simulink model "eBikeDigitalTwin"  (R2023b)
settings: Solver=VariableStepAuto  StartTime=0.0  StopTime=10.0  RelTol=1e-3
libraries: ee_lib x14, fl_lib x7, batteryecm_lib x4, spsPermanentMagnetSynchronousMachineLib x1
settings Model: Creator=epier  LastModifiedBy=epier

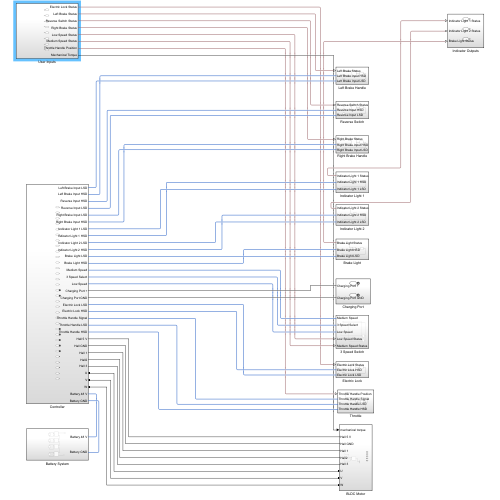
[thumbnail: Simulink's stored preview of the top-level diagram]
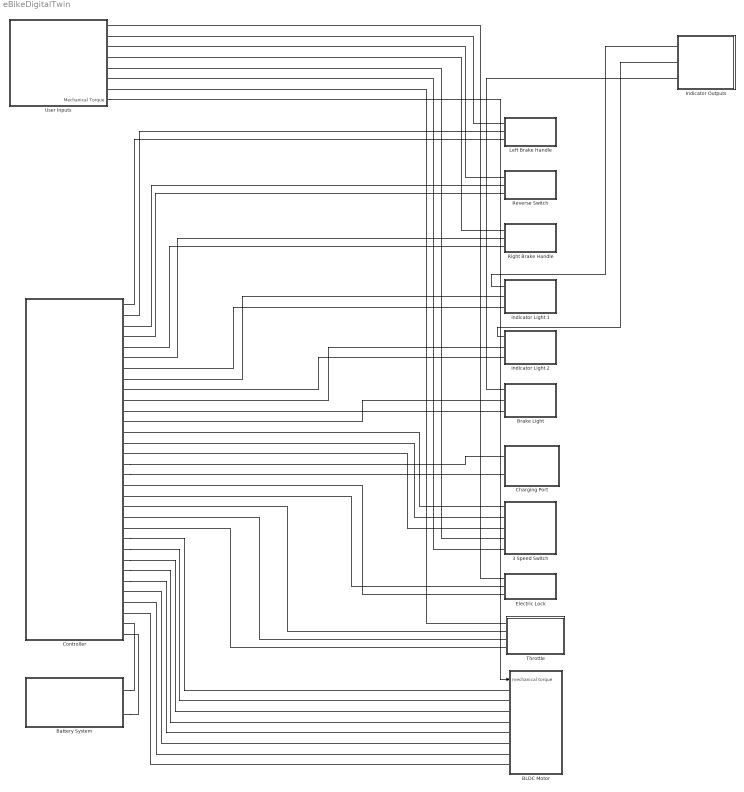
== system eBikeDigitalTwin ==
  3 Speed Switch : Subsystem
  BLDC Motor : Subsystem
      settings: PortSchema="{\"entries\":[{\"content\":{\"sides\":[{\"content\":{},\"type\":\"ConnectorPlacement.EquallySpacedRectSide\",\"uuid\":\"6f305cfd-3a6e-4ac1-8ccb-5bca266a502d\"},{\"content\":{\"connectorIds\":[\"In1\",\"RConn1\",\"RConn2\",\"RConn3\",\"RConn4\",\"RConn5\",\"RConn6\",\"RConn7\",\"RConn8\"],\"side\":\"RIGHT\"},\"type\":\"ConnectorPlacement.EquallySpacedRectSide\",\"uuid\":\"3c37ef43-0ddf-4dcc-b8e6-a30a230bdb34\"},{\"content\":{\"side\":\"TOP\"},\"type\":\"ConnectorPlacement.EquallySpacedRectSide\",\"uuid\":\"8af75aaf-b5e7-47d0-9c7f-87a962c63755\"}]},\"type\":\"ConnectorPlacement.EquallySpacedConnector\",\"uuid\":\"baf254ef-54e0-4d0e-9512-c63c4e1739b8\"}],\"packageUris\":[\"http://schema.mathworks.com/mf0/Connector/R2020b\"],\"version\":\"1.0\"}"
  Battery System : Subsystem
  Brake Light : Subsystem
  Charging Port : Subsystem
  Controller : Subsystem
  Electric Lock : Subsystem
  Indicator Light 1 : Subsystem
  Indicator Light 2 : Subsystem
  Indicator Outputs : Subsystem
  Left Brake Handle : Subsystem
  Reverse Switch : Subsystem
  Right Brake Handle : Subsystem
  Throttle : Subsystem
  User Inputs : Subsystem
      settings: PortSchema="{\"entries\":[{\"content\":{\"sides\":[{\"content\":{},\"type\":\"ConnectorPlacement.EquallySpacedRectSide\",\"uuid\":\"c4874808-4bc0-4391-ab50-9ee5c3ad01f9\"},{\"content\":{\"connectorIds\":[\"RConn1\",\"RConn2\",\"RConn3\",\"RConn4\",\"RConn5\",\"RConn6\",\"RConn7\",\"Out1\"],\"side\":\"RIGHT\"},\"type\":\"ConnectorPlacement.EquallySpacedRectSide\",\"uuid\":\"5fcb0844-4dd2-4d4a-9281-d992b8247c18\"},{\"content\":{\"side\":\"TOP\"},\"type\":\"ConnectorPlacement.EquallySpacedRectSide\",\"uuid\":\"f8d96913-3646-41c7-98dc-9e2b9fe885e6\"}]},\"type\":\"ConnectorPlacement.EquallySpacedConnector\",\"uuid\":\"3c384b36-bf68-40a4-b8b5-a19355291a85\"}],\"packageUris\":[\"http://schema.mathworks.com/mf0/Connector/R2020b\"],\"version\":\"1.0\"}"
  wires:
  User Inputs/1(Mechanical Torque) -> BLDC Motor/1(mechanical torque)
  connections:
  Electric Lock/LConn1 -- User Inputs/RConn1
  Left Brake Handle/LConn1 -- User Inputs/RConn2
  Reverse Switch/LConn1 -- User Inputs/RConn3
  Right Brake Handle/LConn1 -- User Inputs/RConn4
  Left Brake Handle/LConn2 -- Controller/LConn2
  Left Brake Handle/LConn3 -- Controller/LConn1
  Reverse Switch/LConn2 -- Controller/LConn3
  Reverse Switch/LConn3 -- Controller/LConn4
  Right Brake Handle/LConn3 -- Controller/LConn5
  Right Brake Handle/LConn2 -- Controller/LConn6
  Indicator Light 1/LConn1 -- Indicator Outputs/LConn1
  Indicator Light 1/LConn3 -- Controller/LConn7
  Indicator Light 1/LConn2 -- Controller/LConn8
  Indicator Light 2/LConn1 -- Indicator Outputs/LConn2
  Indicator Light 2/LConn3 -- Controller/LConn9
  Indicator Light 2/LConn2 -- Controller/LConn10
  Brake Light/LConn1 -- Indicator Outputs/LConn3
  Brake Light/LConn3 -- Controller/LConn11
  Brake Light/LConn2 -- Controller/LConn12
  3 Speed Switch/LConn4 -- User Inputs/RConn5
  3 Speed Switch/LConn5 -- User Inputs/RConn6
  3 Speed Switch/LConn1 -- Controller/LConn13
  3 Speed Switch/LConn2 -- Controller/LConn14
  3 Speed Switch/LConn3 -- Controller/LConn15
  Electric Lock/LConn3 -- Controller/LConn18
  Electric Lock/LConn2 -- Controller/LConn19
  Throttle/LConn1 -- User Inputs/RConn7
  Throttle/LConn2 -- Controller/LConn20
  Throttle/LConn3 -- Controller/LConn21
  Throttle/LConn4 -- Controller/LConn22
  BLDC Motor/RConn6 -- Controller/LConn28
  BLDC Motor/RConn7 -- Controller/LConn29
  BLDC Motor/RConn8 -- Controller/LConn30
  Controller/LConn23 -- BLDC Motor/RConn1
  Controller/LConn24 -- BLDC Motor/RConn2
  Controller/LConn25 -- BLDC Motor/RConn3
  Controller/LConn26 -- BLDC Motor/RConn4
  Controller/LConn27 -- BLDC Motor/RConn5
  Controller/LConn16 -- Charging Port/LConn1
  Controller/LConn17 -- Charging Port/LConn2
  Battery System/RConn1 -- Controller/LConn31
  Battery System/RConn2 -- Controller/LConn32

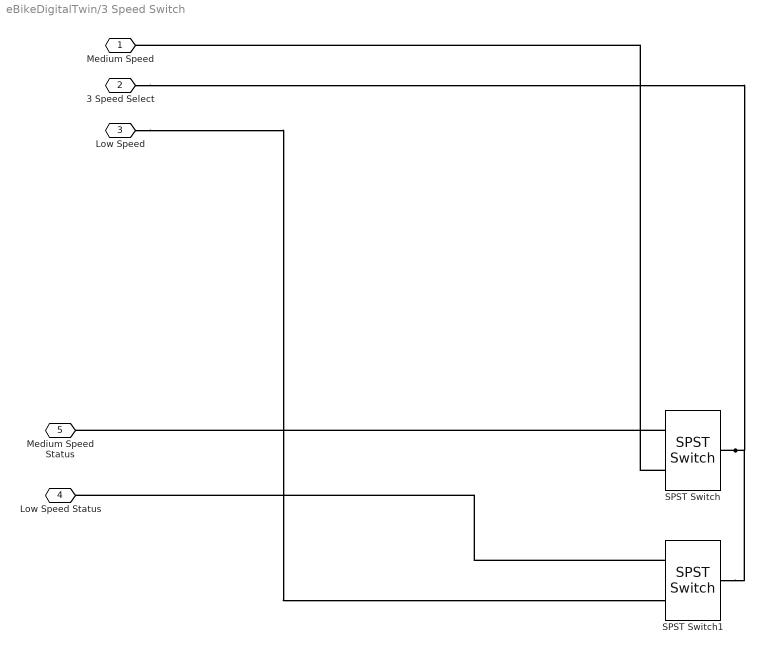
== system eBikeDigitalTwin/3 Speed Switch ==
  SPST Switch : ee_lib/Switches & Breakers/SPST Switch  R_closed=0.01 Ohm  G_open=1e-6 S  Threshold=0.5 V  Width=0 V  model_dynamics=0  t_on=1e-3 s  t_off=1e-3 s  initial_vT=0 V
      settings: InternalSimscapePortConfiguration="{\"Bottom\":[],\"Left\":[{\"id\":\"vT\",\"label\":\"vT\",\"type\":\"input\"},{\"id\":\"p\",\"label\":\"\",\"type\":\"foundation.electrical.electrical\"}],\"Right\":[{\"id\":\"n\",\"label\":\"\",\"type\":\"foundation.electrical.electrical\"}],\"Top\":[]}"
  SPST Switch1 : ee_lib/Switches & Breakers/SPST Switch  R_closed=0.01 Ohm  G_open=1e-6 S  Threshold=0.5 V  Width=0 V  model_dynamics=0  t_on=1e-3 s  t_off=1e-3 s  initial_vT=0 V
      settings: InternalSimscapePortConfiguration="{\"Bottom\":[],\"Left\":[{\"id\":\"vT\",\"label\":\"vT\",\"type\":\"input\"},{\"id\":\"p\",\"label\":\"\",\"type\":\"foundation.electrical.electrical\"}],\"Right\":[{\"id\":\"n\",\"label\":\"\",\"type\":\"foundation.electrical.electrical\"}],\"Top\":[]}"
  Medium Speed : PMIOPort  Side=Left
  3 Speed Select : PMIOPort  Port=2  Side=Left
  Low Speed : PMIOPort  Port=3  Side=Left
  Low Speed Status : PMIOPort  Port=4  Side=Left
  Medium Speed Status : PMIOPort  Port=5  Side=Left
  connections:
  SPST Switch/RConn1 -- 3 Speed Select/RConn1 -- SPST Switch1/RConn1
  SPST Switch1/LConn1 -- Low Speed Status/RConn1
  Low Speed/RConn1 -- SPST Switch1/LConn2
  SPST Switch/LConn1 -- Medium Speed Status/RConn1
  SPST Switch/LConn2 -- Medium Speed/RConn1

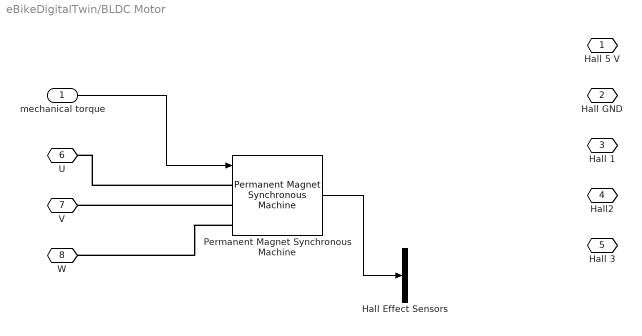
== system eBikeDigitalTwin/BLDC Motor ==
  mechanical torque : Inport
  Hall Effect Sensors : Demux  Outputs=3
  Permanent Magnet Synchronous Machine : spsPermanentMagnetSynchronousMachineLib/Permanent Magnet Synchronous Machine  NbPhases=3  FluxDistribution=Sinusoidal  RotorType=Round  MechanicalLoad=Torque Tm  PresetModel=No  ShowDetailedParameters=on  MeasurementBus=off  Resistance=0.0485  Inductance=8.5e-3  dqInductances=[8.5e-3,8.5e-3]  La=0.000395  MachineConstant=Flux linkage established by magnets (V.s)  Flux=0.1194  VoltageCst=86.6271  TorqueCst=0.7164  Flat=120  Mechanical=[0.0027 0.0004924 4 0]  PolePairs=4  InitialConditions=[0,0, 0,0]  InitialConditions5ph=[0 0 0 0 0 0]  RefAngle=90 degrees behind phase A axis (modified Park)  IterativeDiscreteModel=Trapezoidal non iterative  TsBlock=-1  TsPowergui=0
  Hall 5 V : PMIOPort  Side=Right
  Hall GND : PMIOPort  Port=2  Side=Right
  Hall 1 : PMIOPort  Port=3  Side=Right
  Hall2 : PMIOPort  Port=4  Side=Right
  Hall 3 : PMIOPort  Port=5  Side=Right
  U : PMIOPort  Port=6  Side=Right
  V : PMIOPort  Port=7  Side=Right
  W : PMIOPort  Port=8  Side=Right
  wires:
  Permanent Magnet Synchronous Machine/1 -> Hall Effect Sensors/1
  mechanical torque/1 -> Permanent Magnet Synchronous Machine/1
  connections:
  Permanent Magnet Synchronous Machine/LConn1 -- U/RConn1
  Permanent Magnet Synchronous Machine/LConn2 -- V/RConn1
  Permanent Magnet Synchronous Machine/LConn3 -- W/RConn1

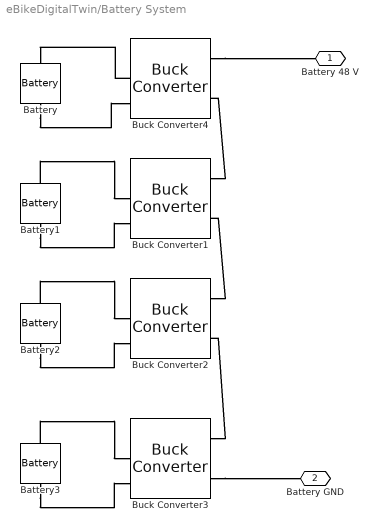
== system eBikeDigitalTwin/Battery System ==
  Battery{,1..3} (4 alike) : batteryecm_lib/Battery  Vnom=12 V  prm_dir=simscape.enum.battery.prm_dir.disabled  R1_dis=2 Ohm  R1_ch=2 Ohm  R1=2 Ohm  prm_AH=simscape.enum.battery.prm_AH.infinite  AH=50 A*hr  V1=11.5 V  AH1=25 A*hr  prm_R2=simscape.enum.battery.prm_R2.disabled  R2=2000 Ohm  Tmeas=298.15 K  charge_measurement_port=simscape.enum.battery.enable.no  prm_dyn=simscape.enum.battery.prm_dyn.off  Rp1=0.005 Ohm  tau1=30 s  Rp2=0.005 Ohm  tau2=30 s  Rp3=0.005 Ohm  tau3=30 s  Rp4=0.005 Ohm  tau4=30 s  Rp5=0.005 Ohm  tau5=30 s  prm_fade=simscape.enum.battery.prm_fade.disabled  N_fade=100  AH_fade=45 A*hr  R1_fade=2.02 Ohm  R1_ch_fade=2.02 Ohm  V1_fade=10.35 V  prm_age=simscape.enum.battery.prm_age.disabled  prm_age_OCV=simscape.enum.battery.prm_age_OCV.OCV  OCV_age=0.9  SOC_age=60  Tmeas_age=298.15 K  delta_time_age_vec=[0] d  temperature_age_vec=[273] K  OCV_scaling_age=2.2134e6  OCV_offset_age=1.632e6  temp_exp_age=0.515833569 V  t_exp_age=0.75  Vnom_T2=12 V  R1_T2=2.2 Ohm  R1_T2_dis=2.2 Ohm  R1_T2_ch=2.2 Ohm  V1_T2=11.4 V  R2_T2=2200 Ohm  Rp1_T2=0.005 Ohm  tau1_T2=30 s  Rp2_T2=0.005 Ohm  tau2_T2=30 s  Rp3_T2=0.005 Ohm  tau3_T2=30 s  Rp4_T2=0.005 Ohm  tau4_T2=30 s  Rp5_T2=0.005 Ohm  tau5_T2=30 s  Tmeas2=273.15 K  thermal_port=simscape.enum.thermaleffects.omit  thermal_mass=30000 J/K  i_specify=off  i_priority=None  i=0 A  i_nominal_specify=off  i_nominal_unit=A  i_nominal_value=1  v_specify=off  v_priority=None  v=0 V  v_nominal_specify=off  v_nominal_unit=V  v_nominal_value=1  charge_specify=off  charge_priority=High  charge=50 A*hr  charge_nominal_specify=off  charge_nominal_unit=A*hr  charge_nominal_value=1  num_cycles_specify=off  num_cycles_priority=High  num_cycles=0  num_cycles_nominal_specify=off  num_cycles_nominal_unit=1  num_cycles_nominal_value=1  temperature_specify=off  temperature_priority=High  temperature=298.15 K  temperature_nominal_specify=off  temperature_nominal_unit=K  temperature_nominal_value=1
  Buck Converter{1..4} (4 alike) : ee_lib/Semiconductors & Converters/Converters/Buck Converter  port_option=ee.enum.controlport.ps  device_type=ee.enum.converters.switchingdevice.ideal  Vf=0.8 V  Ron=0.001 Ohm  Rds=0.001 Ohm  Goff=1e-5 1/Ohm  Vgt=1 V  Vgt_off=-1 V  Ih=1 A  Vth=12 V  K=0  diode_param=ee.enum.converters.protectiondiode.nodynamics  diode_Vf=0.8 V  diode_Ron=0.001 Ohm  diode_Goff=1e-5 1/Ohm  diode_C=50 nF  diode_iRM=-235 A  diode_iF=300 A  diode_idot=-50 A/us  diode_trr_param=ee.enum.converters.diodetrr.trr_factor  diode_trr_factor=3  diode_trr=15 us  diode_Qrr=1500 s*uA  Lf=1e-6 H  Rl=0 Ohm  Cf=1e-7 F  Rf=1e-6 Ohm  snubber_type=ee.enum.converters.snubber.exclude  Cs=1e-7 F  Rs=0.1 Ohm  iL_specify=off  iL_priority=High  iL=0 A  iL_nominal_specify=off  iL_nominal_unit=A  iL_nominal_value=1  vc_specify=off  vc_priority=High  vc=0 V  vc_nominal_specify=off  vc_nominal_unit=V  vc_nominal_value=1
      settings: InternalSimscapePortConfiguration="{\"Bottom\":[],\"Left\":[{\"id\":\"G\",\"label\":\"G\",\"type\":\"input\"},{\"id\":\"p1\",\"label\":\"1+\",\"type\":\"foundation.electrical.electrical\"},{\"id\":\"n1\",\"label\":\"1-\",\"type\":\"foundation.electrical.electrical\"}],\"Right\":[{\"id\":\"p2\",\"label\":\"2+\",\"type\":\"foundation.electrical.electrical\"},{\"id\":\"n2\",\"label\":\"2-\",\"type\":\"foundation.electrical.electrical\"}],\"Top\":[]}"
  Battery 48 V : PMIOPort  Side=Right
  Battery GND : PMIOPort  Port=2  Side=Right
  connections:
  Buck Converter4/LConn2 -- Battery/LConn1
  Battery1/LConn1 -- Buck Converter1/LConn2
  Battery/RConn1 -- Buck Converter4/LConn3
  Buck Converter4/RConn1 -- Battery 48 V/RConn1
  Battery1/RConn1 -- Buck Converter1/LConn3
  Battery2/RConn1 -- Buck Converter2/LConn3
  Battery2/LConn1 -- Buck Converter2/LConn2
  Battery3/RConn1 -- Buck Converter3/LConn3
  Battery3/LConn1 -- Buck Converter3/LConn2
  Buck Converter3/RConn2 -- Battery GND/RConn1
  Buck Converter3/RConn1 -- Buck Converter2/RConn2
  Buck Converter2/RConn1 -- Buck Converter1/RConn2
  Buck Converter1/RConn1 -- Buck Converter4/RConn2

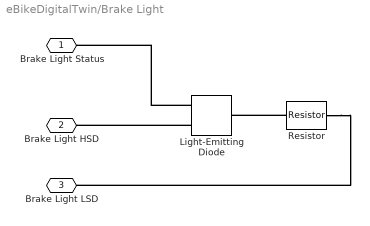
== system eBikeDigitalTwin/Brake Light ==
  Light-Emitting Diode : ee_lib/Sensors & Transducers/Light-Emitting Diode  Gain=0.005 W/A  prmExp=1  I12=[.0017, .003] A  V12=[.9, 1.05] V  IS=5e-5 A  ec=10  RS=0.1 Ohm  Tmeas=25 degC  C_param=1  CJ=20 pF  CJ0=20 pF  VJ=1 V  Mgrad=0.5  Vvec=[.1, 10, 100] V  Cvec=[15, 10, 2] pF  FC=0.5  T_param=1  IS_T2=1.8e-4 A  I1_T2=0.0034 A  V1_T2=1.05 V  Tmeas2=125 degC  EG_param=1  EG=1.11 eV  XTI_param=1  XTI=3  Tdevice=25 degC  i_specify=off  i_priority=None  i=0 A  i_nominal_specify=off  i_nominal_unit=A  i_nominal_value=1  v_specify=off  v_priority=None  v=0 V  v_nominal_specify=off  v_nominal_unit=V  v_nominal_value=1  v_capacitor_specify=off  v_capacitor_priority=High  v_capacitor=0 V  v_capacitor_nominal_specify=off  v_capacitor_nominal_unit=V  v_capacitor_nominal_value=1  thermal_network_parameterization=ee.enum.thermalNetworkTopology.junctionCase  Rth=[0, 10] K/W  Rth_Cauer=[1, 3, 10] K/W  Rth_Foster=[4, 6] K/W  thermal_mass_parameterization=ee.enum.thermalNetwork.timeconstant  thermal_mass=[0, 1] J/K  thermal_mass_Cauer=[1.5, 2, 3] J/K  thermal_mass_Foster=[1.5, 3] J/K  thermal_time_constant=[0, 10] s  thermal_time_constant_Cauer=[1, 3, 10] s  thermal_time_constant_Foster=[6, 18] s  thermal_mass_initial_temperatures=[25, 25] degC  thermal_mass_initial_temperatures_Cauer=[25, 25, 25] degC  steadyState_Foster=simscape.enum.onoff.on  Tvec_initial_Foster=[25, 25, 25, 25] degC
      settings: InternalSimscapePortConfiguration="{\"Bottom\":[],\"Left\":[{\"id\":\"W\",\"label\":\"W\",\"type\":\"output\"},{\"id\":\"p\",\"label\":\"\",\"type\":\"foundation.electrical.electrical\"}],\"Right\":[{\"id\":\"n\",\"label\":\"\",\"type\":\"foundation.electrical.electrical\"}],\"Top\":[]}"
  Resistor : fl_lib/Electrical/Electrical Elements/Resistor  R=1 Ohm  i_specify=off  i_priority=None  i=0 A  i_nominal_specify=off  i_nominal_unit=A  i_nominal_value=1  v_specify=off  v_priority=None  v=0 V  v_nominal_specify=off  v_nominal_unit=V  v_nominal_value=1
  Brake Light Status : PMIOPort  Side=Left
  Brake Light HSD : PMIOPort  Port=2  Side=Left
  Brake Light LSD : PMIOPort  Port=3  Side=Left
  connections:
  Light-Emitting Diode/LConn1 -- Brake Light Status/RConn1
  Resistor/RConn1 -- Brake Light LSD/RConn1
  Resistor/LConn1 -- Light-Emitting Diode/RConn1
  Light-Emitting Diode/LConn2 -- Brake Light HSD/RConn1

== system eBikeDigitalTwin/Charging Port ==
  Charging Port + : PMIOPort  Side=Left
  Charging Port GND : PMIOPort  Port=2  Side=Left

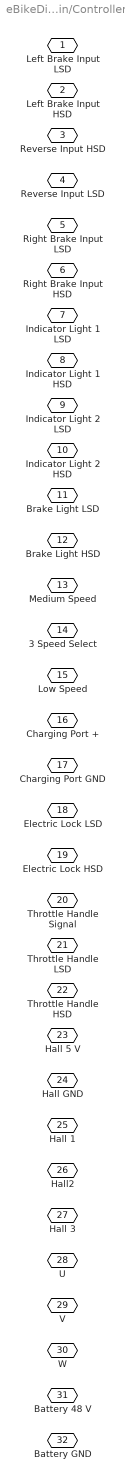
== system eBikeDigitalTwin/Controller ==
  Left Brake Input LSD : PMIOPort  Side=Left
  Left Brake Input HSD : PMIOPort  Port=2  Side=Left
  Reverse Input HSD : PMIOPort  Port=3  Side=Left
  Reverse Input LSD : PMIOPort  Port=4  Side=Left
  Right Brake Input LSD : PMIOPort  Port=5  Side=Left
  Right Brake Input HSD : PMIOPort  Port=6  Side=Left
  Indicator Light 1 LSD : PMIOPort  Port=7  Side=Left
  Indicator Light 1 HSD : PMIOPort  Port=8  Side=Left
  Indicator Light 2 LSD : PMIOPort  Port=9  Side=Left
  Indicator Light 2 HSD : PMIOPort  Port=10  Side=Left
  Brake Light LSD : PMIOPort  Port=11  Side=Left
  Brake Light HSD : PMIOPort  Port=12  Side=Left
  Medium Speed : PMIOPort  Port=13  Side=Left
  3 Speed Select : PMIOPort  Port=14  Side=Left
  Low Speed : PMIOPort  Port=15  Side=Left
  Charging Port + : PMIOPort  Port=16  Side=Left
  Charging Port GND : PMIOPort  Port=17  Side=Left
  Electric Lock LSD : PMIOPort  Port=18  Side=Left
  Electric Lock HSD : PMIOPort  Port=19  Side=Left
  Throttle Handle Signal : PMIOPort  Port=20  Side=Left
  Throttle Handle LSD : PMIOPort  Port=21  Side=Left
  Throttle Handle HSD : PMIOPort  Port=22  Side=Left
  Hall 5 V : PMIOPort  Port=23  Side=Left
  Hall GND : PMIOPort  Port=24  Side=Left
  Hall 1 : PMIOPort  Port=25  Side=Left
  Hall2 : PMIOPort  Port=26  Side=Left
  Hall 3 : PMIOPort  Port=27  Side=Left
  U : PMIOPort  Port=28  Side=Left
  V : PMIOPort  Port=29  Side=Left
  W : PMIOPort  Port=30  Side=Left
  Battery 48 V : PMIOPort  Port=31  Side=Left
  Battery GND : PMIOPort  Port=32  Side=Left

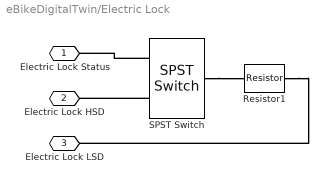
== system eBikeDigitalTwin/Electric Lock ==
  Resistor1 : fl_lib/Electrical/Electrical Elements/Resistor  R=0.8 Ohm  i_specify=off  i_priority=None  i=0 A  i_nominal_specify=off  i_nominal_unit=A  i_nominal_value=1  v_specify=off  v_priority=None  v=0 V  v_nominal_specify=off  v_nominal_unit=V  v_nominal_value=1
  SPST Switch : ee_lib/Switches & Breakers/SPST Switch  R_closed=0.01 Ohm  G_open=1e-6 S  Threshold=0.5 V  Width=0 V  model_dynamics=0  t_on=1e-3 s  t_off=1e-3 s  initial_vT=0 V
      settings: InternalSimscapePortConfiguration="{\"Bottom\":[],\"Left\":[{\"id\":\"vT\",\"label\":\"vT\",\"type\":\"input\"},{\"id\":\"p\",\"label\":\"\",\"type\":\"foundation.electrical.electrical\"}],\"Right\":[{\"id\":\"n\",\"label\":\"\",\"type\":\"foundation.electrical.electrical\"}],\"Top\":[]}"
  Electric Lock Status : PMIOPort  Side=Left
  Electric Lock HSD : PMIOPort  Port=2  Side=Left
  Electric Lock LSD : PMIOPort  Port=3  Side=Left
  connections:
  SPST Switch/RConn1 -- Resistor1/LConn1
  SPST Switch/LConn1 -- Electric Lock Status/RConn1
  Resistor1/RConn1 -- Electric Lock LSD/RConn1
  SPST Switch/LConn2 -- Electric Lock HSD/RConn1

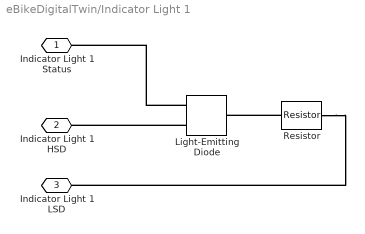
== system eBikeDigitalTwin/Indicator Light 1 ==
  Light-Emitting Diode : ee_lib/Sensors & Transducers/Light-Emitting Diode  Gain=0.005 W/A  prmExp=1  I12=[.0017, .003] A  V12=[.9, 1.05] V  IS=5e-5 A  ec=10  RS=0.1 Ohm  Tmeas=25 degC  C_param=1  CJ=20 pF  CJ0=20 pF  VJ=1 V  Mgrad=0.5  Vvec=[.1, 10, 100] V  Cvec=[15, 10, 2] pF  FC=0.5  T_param=1  IS_T2=1.8e-4 A  I1_T2=0.0034 A  V1_T2=1.05 V  Tmeas2=125 degC  EG_param=1  EG=1.11 eV  XTI_param=1  XTI=3  Tdevice=25 degC  i_specify=off  i_priority=None  i=0 A  i_nominal_specify=off  i_nominal_unit=A  i_nominal_value=1  v_specify=off  v_priority=None  v=0 V  v_nominal_specify=off  v_nominal_unit=V  v_nominal_value=1  v_capacitor_specify=off  v_capacitor_priority=High  v_capacitor=0 V  v_capacitor_nominal_specify=off  v_capacitor_nominal_unit=V  v_capacitor_nominal_value=1  thermal_network_parameterization=ee.enum.thermalNetworkTopology.junctionCase  Rth=[0, 10] K/W  Rth_Cauer=[1, 3, 10] K/W  Rth_Foster=[4, 6] K/W  thermal_mass_parameterization=ee.enum.thermalNetwork.timeconstant  thermal_mass=[0, 1] J/K  thermal_mass_Cauer=[1.5, 2, 3] J/K  thermal_mass_Foster=[1.5, 3] J/K  thermal_time_constant=[0, 10] s  thermal_time_constant_Cauer=[1, 3, 10] s  thermal_time_constant_Foster=[6, 18] s  thermal_mass_initial_temperatures=[25, 25] degC  thermal_mass_initial_temperatures_Cauer=[25, 25, 25] degC  steadyState_Foster=simscape.enum.onoff.on  Tvec_initial_Foster=[25, 25, 25, 25] degC
      settings: InternalSimscapePortConfiguration="{\"Bottom\":[],\"Left\":[{\"id\":\"W\",\"label\":\"W\",\"type\":\"output\"},{\"id\":\"p\",\"label\":\"\",\"type\":\"foundation.electrical.electrical\"}],\"Right\":[{\"id\":\"n\",\"label\":\"\",\"type\":\"foundation.electrical.electrical\"}],\"Top\":[]}"
  Resistor : fl_lib/Electrical/Electrical Elements/Resistor  R=1 Ohm  i_specify=off  i_priority=None  i=0 A  i_nominal_specify=off  i_nominal_unit=A  i_nominal_value=1  v_specify=off  v_priority=None  v=0 V  v_nominal_specify=off  v_nominal_unit=V  v_nominal_value=1
  Indicator Light 1 Status : PMIOPort  Side=Left
  Indicator Light 1 HSD : PMIOPort  Port=2  Side=Left
  Indicator Light 1 LSD : PMIOPort  Port=3  Side=Left
  connections:
  Light-Emitting Diode/LConn1 -- Indicator Light 1 Status/RConn1
  Resistor/RConn1 -- Indicator Light 1 LSD/RConn1
  Resistor/LConn1 -- Light-Emitting Diode/RConn1
  Light-Emitting Diode/LConn2 -- Indicator Light 1 HSD/RConn1

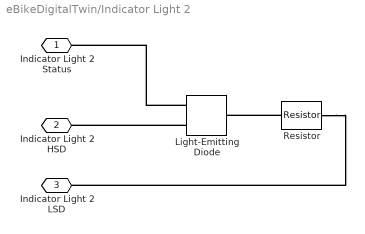
== system eBikeDigitalTwin/Indicator Light 2 ==
  Light-Emitting Diode : ee_lib/Sensors & Transducers/Light-Emitting Diode  Gain=0.005 W/A  prmExp=1  I12=[.0017, .003] A  V12=[.9, 1.05] V  IS=5e-5 A  ec=10  RS=0.1 Ohm  Tmeas=25 degC  C_param=1  CJ=20 pF  CJ0=20 pF  VJ=1 V  Mgrad=0.5  Vvec=[.1, 10, 100] V  Cvec=[15, 10, 2] pF  FC=0.5  T_param=1  IS_T2=1.8e-4 A  I1_T2=0.0034 A  V1_T2=1.05 V  Tmeas2=125 degC  EG_param=1  EG=1.11 eV  XTI_param=1  XTI=3  Tdevice=25 degC  i_specify=off  i_priority=None  i=0 A  i_nominal_specify=off  i_nominal_unit=A  i_nominal_value=1  v_specify=off  v_priority=None  v=0 V  v_nominal_specify=off  v_nominal_unit=V  v_nominal_value=1  v_capacitor_specify=off  v_capacitor_priority=High  v_capacitor=0 V  v_capacitor_nominal_specify=off  v_capacitor_nominal_unit=V  v_capacitor_nominal_value=1  thermal_network_parameterization=ee.enum.thermalNetworkTopology.junctionCase  Rth=[0, 10] K/W  Rth_Cauer=[1, 3, 10] K/W  Rth_Foster=[4, 6] K/W  thermal_mass_parameterization=ee.enum.thermalNetwork.timeconstant  thermal_mass=[0, 1] J/K  thermal_mass_Cauer=[1.5, 2, 3] J/K  thermal_mass_Foster=[1.5, 3] J/K  thermal_time_constant=[0, 10] s  thermal_time_constant_Cauer=[1, 3, 10] s  thermal_time_constant_Foster=[6, 18] s  thermal_mass_initial_temperatures=[25, 25] degC  thermal_mass_initial_temperatures_Cauer=[25, 25, 25] degC  steadyState_Foster=simscape.enum.onoff.on  Tvec_initial_Foster=[25, 25, 25, 25] degC
      settings: InternalSimscapePortConfiguration="{\"Bottom\":[],\"Left\":[{\"id\":\"W\",\"label\":\"W\",\"type\":\"output\"},{\"id\":\"p\",\"label\":\"\",\"type\":\"foundation.electrical.electrical\"}],\"Right\":[{\"id\":\"n\",\"label\":\"\",\"type\":\"foundation.electrical.electrical\"}],\"Top\":[]}"
  Resistor : fl_lib/Electrical/Electrical Elements/Resistor  R=1 Ohm  i_specify=off  i_priority=None  i=0 A  i_nominal_specify=off  i_nominal_unit=A  i_nominal_value=1  v_specify=off  v_priority=None  v=0 V  v_nominal_specify=off  v_nominal_unit=V  v_nominal_value=1
  Indicator Light 2 Status : PMIOPort  Side=Left
  Indicator Light 2 HSD : PMIOPort  Port=2  Side=Left
  Indicator Light 2 LSD : PMIOPort  Port=3  Side=Left
  connections:
  Light-Emitting Diode/LConn1 -- Indicator Light 2 Status/RConn1
  Resistor/RConn1 -- Indicator Light 2 LSD/RConn1
  Resistor/LConn1 -- Light-Emitting Diode/RConn1
  Light-Emitting Diode/LConn2 -- Indicator Light 2 HSD/RConn1

== system eBikeDigitalTwin/Indicator Outputs ==
  Indicator Light 1 Status : PMIOPort  Side=Left
  Indicator Light 2 Status : PMIOPort  Port=2  Side=Left
  Brake Light Status : PMIOPort  Port=3  Side=Left

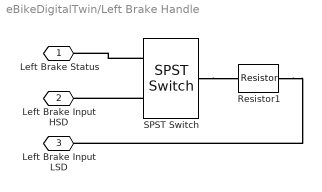
== system eBikeDigitalTwin/Left Brake Handle ==
  Resistor1 : fl_lib/Electrical/Electrical Elements/Resistor  R=0.8 Ohm  i_specify=off  i_priority=None  i=0 A  i_nominal_specify=off  i_nominal_unit=A  i_nominal_value=1  v_specify=off  v_priority=None  v=0 V  v_nominal_specify=off  v_nominal_unit=V  v_nominal_value=1
  SPST Switch : ee_lib/Switches & Breakers/SPST Switch  R_closed=0.01 Ohm  G_open=1e-6 S  Threshold=0.5 V  Width=0 V  model_dynamics=0  t_on=1e-3 s  t_off=1e-3 s  initial_vT=0 V
      settings: InternalSimscapePortConfiguration="{\"Bottom\":[],\"Left\":[{\"id\":\"vT\",\"label\":\"vT\",\"type\":\"input\"},{\"id\":\"p\",\"label\":\"\",\"type\":\"foundation.electrical.electrical\"}],\"Right\":[{\"id\":\"n\",\"label\":\"\",\"type\":\"foundation.electrical.electrical\"}],\"Top\":[]}"
  Left Brake Status : PMIOPort  Side=Left
  Left Brake Input HSD : PMIOPort  Port=2  Side=Left
  Left Brake Input LSD : PMIOPort  Port=3  Side=Left
  connections:
  SPST Switch/RConn1 -- Resistor1/LConn1
  SPST Switch/LConn1 -- Left Brake Status/RConn1
  Resistor1/RConn1 -- Left Brake Input LSD/RConn1
  SPST Switch/LConn2 -- Left Brake Input HSD/RConn1

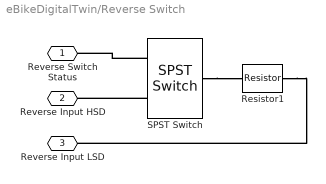
== system eBikeDigitalTwin/Reverse Switch ==
  Resistor1 : fl_lib/Electrical/Electrical Elements/Resistor  R=0.8 Ohm  i_specify=off  i_priority=None  i=0 A  i_nominal_specify=off  i_nominal_unit=A  i_nominal_value=1  v_specify=off  v_priority=None  v=0 V  v_nominal_specify=off  v_nominal_unit=V  v_nominal_value=1
  SPST Switch : ee_lib/Switches & Breakers/SPST Switch  R_closed=0.01 Ohm  G_open=1e-6 S  Threshold=0.5 V  Width=0 V  model_dynamics=0  t_on=1e-3 s  t_off=1e-3 s  initial_vT=0 V
      settings: InternalSimscapePortConfiguration="{\"Bottom\":[],\"Left\":[{\"id\":\"vT\",\"label\":\"vT\",\"type\":\"input\"},{\"id\":\"p\",\"label\":\"\",\"type\":\"foundation.electrical.electrical\"}],\"Right\":[{\"id\":\"n\",\"label\":\"\",\"type\":\"foundation.electrical.electrical\"}],\"Top\":[]}"
  Reverse Switch Status : PMIOPort  Side=Left
  Reverse Input HSD : PMIOPort  Port=2  Side=Left
  Reverse Input LSD : PMIOPort  Port=3  Side=Left
  connections:
  SPST Switch/RConn1 -- Resistor1/LConn1
  SPST Switch/LConn1 -- Reverse Switch Status/RConn1
  Resistor1/RConn1 -- Reverse Input LSD/RConn1
  SPST Switch/LConn2 -- Reverse Input HSD/RConn1

== system eBikeDigitalTwin/Right Brake Handle ==
  Resistor1 : fl_lib/Electrical/Electrical Elements/Resistor  R=0.8 Ohm  i_specify=off  i_priority=None  i=0 A  i_nominal_specify=off  i_nominal_unit=A  i_nominal_value=1  v_specify=off  v_priority=None  v=0 V  v_nominal_specify=off  v_nominal_unit=V  v_nominal_value=1
  SPST Switch : ee_lib/Switches & Breakers/SPST Switch  R_closed=0.01 Ohm  G_open=1e-6 S  Threshold=0.5 V  Width=0 V  model_dynamics=0  t_on=1e-3 s  t_off=1e-3 s  initial_vT=0 V
      settings: InternalSimscapePortConfiguration="{\"Bottom\":[],\"Left\":[{\"id\":\"vT\",\"label\":\"vT\",\"type\":\"input\"},{\"id\":\"p\",\"label\":\"\",\"type\":\"foundation.electrical.electrical\"}],\"Right\":[{\"id\":\"n\",\"label\":\"\",\"type\":\"foundation.electrical.electrical\"}],\"Top\":[]}"
  Right Brake Input HSD : PMIOPort  Port=2  Side=Left
  Right Brake Status : PMIOPort  Side=Left
  Right Brake Input LSD : PMIOPort  Port=3  Side=Left
  connections:
  SPST Switch/RConn1 -- Resistor1/LConn1
  SPST Switch/LConn1 -- Right Brake Status/RConn1
  Resistor1/RConn1 -- Right Brake Input LSD/RConn1
  SPST Switch/LConn2 -- Right Brake Input HSD/RConn1

== system eBikeDigitalTwin/Throttle ==
  Potentiometer : ee_lib/Passive/Potentiometer  nPorts=ee.enum.passive.potentiometer.nPorts.Three  R0=1000 Ohm  Rw=1 Ohm  xmin=0  xmax=1  minResistance=1 Ohm  maxResistance=999 Ohm  xmin2port=0  xmax2port=1  Taper=ee.enum.passive.potentiometer.linOrLog.lin  Rcenter=200 Ohm  Gradient=ee.enum.passive.potentiometer.gradient.higherR
      settings: InternalSimscapePortConfiguration="{\"Bottom\":[],\"Left\":[{\"id\":\"pinL\",\"label\":\"L\",\"type\":\"foundation.electrical.electrical\"},{\"id\":\"W\",\"label\":\"W\",\"type\":\"foundation.electrical.electrical\"}],\"Right\":[{\"id\":\"pinR\",\"label\":\"R\",\"type\":\"foundation.electrical.electrical\"},{\"id\":\"x\",\"label\":\"x\",\"type\":\"input\"}],\"Top\":[]}"
  Throttle Handle Position : PMIOPort  Side=Left
  Throttle Handle Signal : PMIOPort  Port=2  Side=Left
  Throttle Handle LSD : PMIOPort  Port=3  Side=Left
  Throttle Handle HSD : PMIOPort  Port=4  Side=Left
  connections:
  Potentiometer/RConn1 -- Throttle Handle LSD/RConn1
  Potentiometer/LConn2 -- Throttle Handle Signal/RConn1
  Potentiometer/LConn1 -- Throttle Handle HSD/RConn1
  Potentiometer/RConn2 -- Throttle Handle Position/RConn1

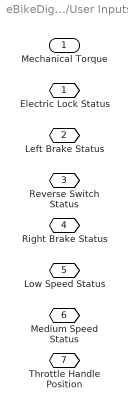
== system eBikeDigitalTwin/User Inputs ==
  Electric Lock Status : PMIOPort  Side=Right
  Left Brake Status : PMIOPort  Port=2  Side=Right
  Reverse Switch Status : PMIOPort  Port=3  Side=Right
  Right Brake Status : PMIOPort  Port=4  Side=Right
  Low Speed Status : PMIOPort  Port=5  Side=Right
  Medium Speed Status : PMIOPort  Port=6  Side=Right
  Throttle Handle Position : PMIOPort  Port=7  Side=Right
  Mechanical Torque : Outport
